simulink model "Discrete_sim"  (R2025a)
settings: Solver=FixedStepDiscrete  StartTime=0.0  StopTime=20  FixedStep=0.1  RelTol=1e-3
settings Model: Creator=user  LastModifiedBy=user

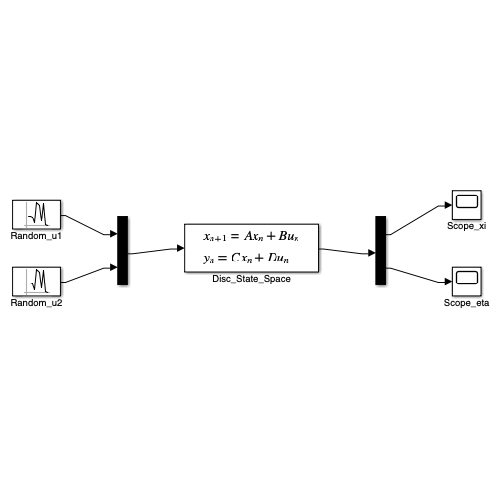
[thumbnail: Simulink's stored preview of the top-level diagram]
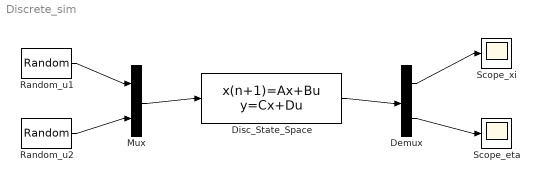
== system Discrete_sim ==
  Demux : Demux  Outputs=2
  Disc_State_Space : DiscreteStateSpace  A=[1 0.0999583385413567 0 -0.00249947921006751;0 0.998750260394966 0 -0.0499791692706783;0 0.00249947921006751 1 0.0999583385413567;0 0.0499791692706783 0 0.998750260394966]  B=[0.00499895842013501 -8.33229172866849e-05;0.0999583385413566 -0.00249947921006751;8.33229172866849e-05 0.00499895842013502;0.00249947921006751 0.0999583385413567]  C=[1 0 0 0;0 0 1 0]  D=[0 0;0 0]  InitialCondition=[0 0.1 0 0.1]  SampleTime=0.1
  Mux : Mux  Inputs=2
  Random_u1 : RandomNumber  SampleTime=0.1
  Random_u2 : RandomNumber  SampleTime=0.1
  Scope_eta : Scope
  Scope_xi : Scope
  wires:
  Random_u1/1 -> Mux/1
  Random_u2/1 -> Mux/2
  Mux/1 -> Disc_State_Space/1
  Disc_State_Space/1 -> Demux/1
  Demux/1 -> Scope_xi/1
  Demux/2 -> Scope_eta/1
